simulink model "Backstepping_control"  (R2020b)
settings: Solver=FixedStepAuto  StartTime=0.0  StopTime=500  FixedStep=1e-3  RelTol=1e-3
values from neighbouring files (symbols this model uses):
  g_par = 9.81    [init.m]
  J_par = (M_par*4*l_par^2)/12    (= 192666666.667)    [init.m]
  l_par = 34    [init.m]
  M_par = 5e5    (= 500000)    [init.m]
  mu_x_par = 0.5*rho_par*cdx_par*Ax_par    (= 152.439)    [init.m]
  mu_y_par = 0.5*rho_par*cdy_par*Ay_par    (= 1.28880775561)    [init.m]
  theta0 = deg2rad(15)    [init.m]
  x0 = 2    [init.m]
  y0 = -5    [init.m]
settings Model: Creator=chiara-s  LastModifiedBy=giorg

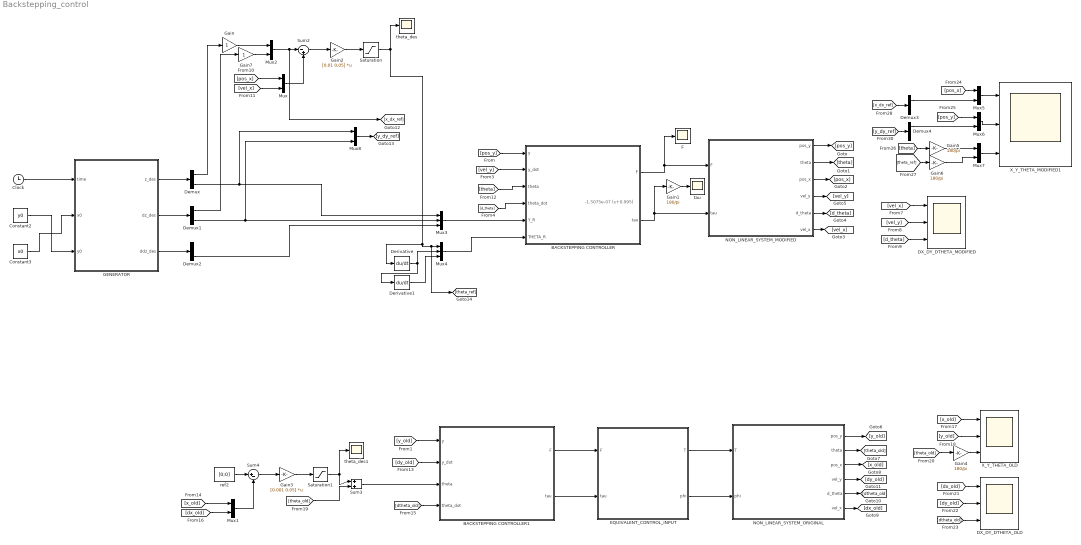
== system Backstepping_control ==
  note: -1.5075e-07 (s+0.995)
  BACKSTEPPING CONTROLLER : Subsystem
  BACKSTEPPING CONTROLLER1 : Subsystem
  Clock : Clock
  Constant2 : Constant  Value=y0
  Constant3 : Constant  Value=x0
  DX_DY_DTHETA_MODIFIED : Scope  NumInputPorts=3
  DX_DY_DTHETA_OLD : Scope  NumInputPorts=3
  Demux{,1..4} (5 alike) : Demux  Outputs=2
  Derivative : Derivative
  Derivative1 : Derivative
  EQUIVALENT_CONTROL_INPUT : MATLAB Function  TreatAsAtomicUnit=on
  F : Scope
  GENERATOR : MATLAB Function  TreatAsAtomicUnit=on
  Gain : Gain
  Gain{1,4..6} (4 alike) : Gain  Gain=180/pi
  Gain2 : Gain  Gain=[0.01 0.05]  Multiplication=Matrix(K*u)
  Gain3 : Gain  Gain=[0.001 0.05]  Multiplication=Matrix(K*u)
  Gain7 : Gain
  Mux{,1..2,5..8} (7 alike) : Mux  Inputs=2
  Mux3 : Mux  Inputs=3
  Mux4 : Mux  Inputs=3
  NON_LINEAR_SYSTEM_MODIFIED : Subsystem
  NON_LINEAR_SYSTEM_ORIGINAL : Subsystem
  Saturation : Saturate  UpperLimit=0.2  LowerLimit=-0.2
  Saturation1 : Saturate  UpperLimit=0.2  LowerLimit=-0.2
  Sum2 : Sum  Inputs=|-+
  Sum3 : Sum  Inputs=|++
  Sum4 : Sum  Inputs=|+-
  X_Y_THETA_MODIFIED1 : Scope  NumInputPorts=3
  X_Y_THETA_OLD : Scope  NumInputPorts=3
  ref2 : Constant  Value=[0;0]
  tau : Scope
  theta_des : Scope
  theta_des1 : Scope
  wires:
  NON_LINEAR_SYSTEM_MODIFIED/1(pos_y) -> [pos_y]
  NON_LINEAR_SYSTEM_MODIFIED/2(theta) -> [theta]
  NON_LINEAR_SYSTEM_MODIFIED/3(pos_x) -> [pos_x]
  NON_LINEAR_SYSTEM_MODIFIED/4(vel_y) -> [vel_y]
  NON_LINEAR_SYSTEM_MODIFIED/5(d_theta) -> [d_theta]
  NON_LINEAR_SYSTEM_MODIFIED/6(vel_x) -> [vel_x]
  [d_theta] -> BACKSTEPPING CONTROLLER/4(theta_dot)
  [pos_y] -> BACKSTEPPING CONTROLLER/1(y)
  [vel_y] -> BACKSTEPPING CONTROLLER/2(y_dot)
  BACKSTEPPING CONTROLLER/1(F) -> NON_LINEAR_SYSTEM_MODIFIED/1(F), F/1
  BACKSTEPPING CONTROLLER/2(tau) -> Gain1/1, NON_LINEAR_SYSTEM_MODIFIED/2(tau)
  [vel_x] -> DX_DY_DTHETA_MODIFIED/1
  [vel_y] -> DX_DY_DTHETA_MODIFIED/2
  [d_theta] -> DX_DY_DTHETA_MODIFIED/3
  Gain1/1 -> tau/1
  Gain2/1 -> Saturation/1
  Mux2/1 -> [x_dx_ref], Sum2/1
  Sum2/1 -> Gain2/1
  Mux/1 -> Sum2/2
  [pos_x] -> Mux/1
  [vel_x] -> Mux/2
  NON_LINEAR_SYSTEM_ORIGINAL/3(pos_x) -> [x_old]
  NON_LINEAR_SYSTEM_ORIGINAL/1(pos_y) -> [y_old]
  NON_LINEAR_SYSTEM_ORIGINAL/4(vel_y) -> [dy_old]
  NON_LINEAR_SYSTEM_ORIGINAL/5(d_theta) -> [dtheta_old]
  NON_LINEAR_SYSTEM_ORIGINAL/2(theta) -> [theta_old]
  NON_LINEAR_SYSTEM_ORIGINAL/6(vel_x) -> [dx_old]
  BACKSTEPPING CONTROLLER1/1(F) -> EQUIVALENT_CONTROL_INPUT/1(F)
  BACKSTEPPING CONTROLLER1/2(tau) -> EQUIVALENT_CONTROL_INPUT/2(tau)
  EQUIVALENT_CONTROL_INPUT/1(T) -> NON_LINEAR_SYSTEM_ORIGINAL/1(T)
  EQUIVALENT_CONTROL_INPUT/2(phi) -> NON_LINEAR_SYSTEM_ORIGINAL/2(phi)
  [y_old] -> BACKSTEPPING CONTROLLER1/1(y)
  [dy_old] -> BACKSTEPPING CONTROLLER1/2(y_dot)
  [dtheta_old] -> BACKSTEPPING CONTROLLER1/4(theta_dot)
  ref2/1 -> Sum4/1
  Sum3/1 -> BACKSTEPPING CONTROLLER1/3(theta)
  [theta_old] -> Sum3/2
  Sum4/1 -> Gain3/1
  [dx_old] -> Mux1/2
  [x_old] -> Mux1/1
  Mux1/1 -> Sum4/2
  Gain3/1 -> Saturation1/1
  Saturation1/1 -> theta_des1/1, Sum3/1
  [x_old] -> X_Y_THETA_OLD/1
  [y_old] -> X_Y_THETA_OLD/2
  [theta_old] -> Gain4/1
  [dx_old] -> DX_DY_DTHETA_OLD/1
  [dy_old] -> DX_DY_DTHETA_OLD/2
  [dtheta_old] -> DX_DY_DTHETA_OLD/3
  Gain4/1 -> X_Y_THETA_OLD/3
  Mux3/1 -> BACKSTEPPING CONTROLLER/5(Y_R)
  Clock/1 -> GENERATOR/1(time)
  Constant2/1 -> GENERATOR/3(y0)
  Constant3/1 -> GENERATOR/2(x0)
  [theta] -> BACKSTEPPING CONTROLLER/3(theta)
  GENERATOR/3(ddz_des) -> Demux2/1
  GENERATOR/2(dz_des) -> Demux1/1
  GENERATOR/1(z_des) -> Demux/1
  Mux4/1 -> BACKSTEPPING CONTROLLER/6(THETA_R)
  Gain6/1 -> Mux7/2
  Mux7/1 -> X_Y_THETA_MODIFIED1/3
  [theta_ref] -> Gain6/1
  Gain5/1 -> Mux7/1
  [x_dx_ref] -> Demux3/1
  Mux6/1 -> X_Y_THETA_MODIFIED1/2
  [pos_x] -> Mux5/1
  Demux3/1 -> Mux5/2
  [pos_y] -> Mux6/1
  [theta] -> Gain5/1
  Mux5/1 -> X_Y_THETA_MODIFIED1/1
  Demux4/1 -> Mux6/2
  [y_dy_ref] -> Demux4/1
  Saturation/1 -> theta_des/1, [theta_ref], Mux4/1, Derivative/1
  Demux/1 -> Gain/1
  Demux1/1 -> Gain7/1
  Derivative/1 -> Mux4/2, Derivative1/1
  Demux/2 -> Mux8/1, Mux3/1
  Demux1/2 -> Mux8/2, Mux3/2
  Demux2/2 -> Mux3/3
  Mux8/1 -> [y_dy_ref]
  Gain/1 -> Mux2/1
  Gain7/1 -> Mux2/2
  Derivative1/1 -> Mux4/3

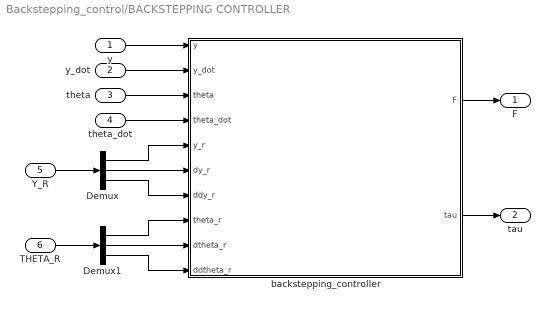
== system Backstepping_control/BACKSTEPPING CONTROLLER ==
  y : Inport
  y_dot : Inport  Port=2
  theta : Inport  Port=3
  theta_dot : Inport  Port=4
  Y_R : Inport  Port=5
  THETA_R : Inport  Port=6
  Demux : Demux  Outputs=3
  Demux1 : Demux  Outputs=3
  backstepping_controller : MATLAB Function  TreatAsAtomicUnit=on
  F : Outport
  tau : Outport  Port=2
  wires:
  backstepping_controller/1(F) -> F/1
  backstepping_controller/2(tau) -> tau/1
  y/1 -> backstepping_controller/1(y)
  y_dot/1 -> backstepping_controller/2(y_dot)
  theta/1 -> backstepping_controller/3(theta)
  theta_dot/1 -> backstepping_controller/4(theta_dot)
  Demux/1 -> backstepping_controller/5(y_r)
  Demux/2 -> backstepping_controller/6(dy_r)
  Demux/3 -> backstepping_controller/7(ddy_r)
  Y_R/1 -> Demux/1
  Demux1/2 -> backstepping_controller/9(dtheta_r)
  Demux1/1 -> backstepping_controller/8(theta_r)
  Demux1/3 -> backstepping_controller/10(ddtheta_r)
  THETA_R/1 -> Demux1/1

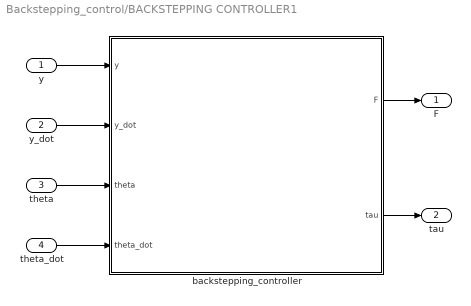
== system Backstepping_control/BACKSTEPPING CONTROLLER1 ==
  y : Inport
  y_dot : Inport  Port=2
  theta : Inport  Port=3
  theta_dot : Inport  Port=4
  backstepping_controller : MATLAB Function  TreatAsAtomicUnit=on
  F : Outport
  tau : Outport  Port=2
  wires:
  backstepping_controller/1(F) -> F/1
  backstepping_controller/2(tau) -> tau/1
  y/1 -> backstepping_controller/1(y)
  y_dot/1 -> backstepping_controller/2(y_dot)
  theta/1 -> backstepping_controller/3(theta)
  theta_dot/1 -> backstepping_controller/4(theta_dot)

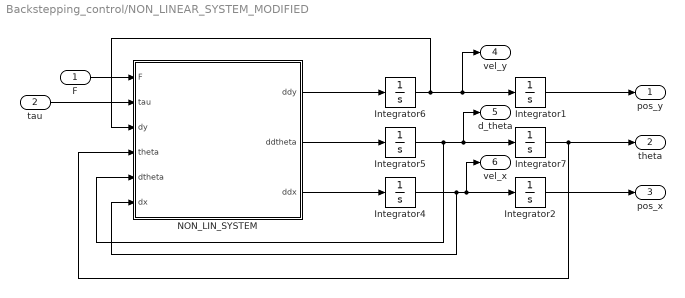
== system Backstepping_control/NON_LINEAR_SYSTEM_MODIFIED ==
  F : Inport
  tau : Inport  Port=2
  Integrator1 : Integrator  InitialCondition=y0
  Integrator2 : Integrator  InitialCondition=x0
  Integrator4 : Integrator
  Integrator5 : Integrator
  Integrator6 : Integrator
  Integrator7 : Integrator  InitialCondition=theta0
  NON_LIN_SYSTEM : MATLAB Function  TreatAsAtomicUnit=on
  pos_y : Outport
  theta : Outport  Port=2
  pos_x : Outport  Port=3
  vel_y : Outport  Port=4
  d_theta : Outport  Port=5
  vel_x : Outport  Port=6
  wires:
  Integrator2/1 -> pos_x/1
  Integrator7/1 -> NON_LIN_SYSTEM/4(theta), theta/1
  NON_LIN_SYSTEM/2(ddtheta) -> Integrator5/1
  tau/1 -> NON_LIN_SYSTEM/2(tau)
  Integrator1/1 -> pos_y/1
  F/1 -> NON_LIN_SYSTEM/1(F)
  Integrator6/1 -> Integrator1/1, vel_y/1, NON_LIN_SYSTEM/3(dy)
  Integrator4/1 -> NON_LIN_SYSTEM/6(dx), vel_x/1, Integrator2/1
  NON_LIN_SYSTEM/1(ddy) -> Integrator6/1
  Integrator5/1 -> NON_LIN_SYSTEM/5(dtheta), Integrator7/1, d_theta/1
  NON_LIN_SYSTEM/3(ddx) -> Integrator4/1

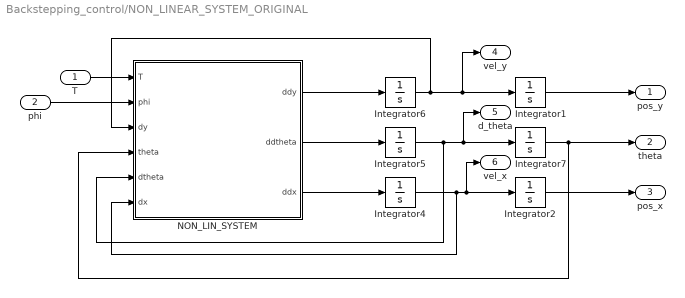
== system Backstepping_control/NON_LINEAR_SYSTEM_ORIGINAL ==
  T : Inport
  phi : Inport  Port=2
  Integrator1 : Integrator  InitialCondition=y0
  Integrator2 : Integrator  InitialCondition=x0
  Integrator4 : Integrator
  Integrator5 : Integrator
  Integrator6 : Integrator
  Integrator7 : Integrator  InitialCondition=theta0
  NON_LIN_SYSTEM : MATLAB Function  TreatAsAtomicUnit=on
  pos_y : Outport
  theta : Outport  Port=2
  pos_x : Outport  Port=3
  vel_y : Outport  Port=4
  d_theta : Outport  Port=5
  vel_x : Outport  Port=6
  wires:
  Integrator2/1 -> pos_x/1
  Integrator7/1 -> NON_LIN_SYSTEM/4(theta), theta/1
  NON_LIN_SYSTEM/2(ddtheta) -> Integrator5/1
  phi/1 -> NON_LIN_SYSTEM/2(phi)
  Integrator1/1 -> pos_y/1
  T/1 -> NON_LIN_SYSTEM/1(T)
  Integrator6/1 -> Integrator1/1, vel_y/1, NON_LIN_SYSTEM/3(dy)
  Integrator4/1 -> NON_LIN_SYSTEM/6(dx), vel_x/1, Integrator2/1
  NON_LIN_SYSTEM/1(ddy) -> Integrator6/1
  Integrator5/1 -> NON_LIN_SYSTEM/5(dtheta), Integrator7/1, d_theta/1
  NON_LIN_SYSTEM/3(ddx) -> Integrator4/1

== matlab function Backstepping_control/GENERATOR ==
  data: time input; x0 input; y0 input; z_des output; dz_des output; ddz_des output
function  [z_des, dz_des, ddz_des] = fcn(time,x0,y0)
t= time;
pos_init = [x0;y0];
z_des = pos_init + [20*sin(0.1*t); 10*sin(0.2*t)];
dz_des = [cos(0.1*t)*2; cos(0.2*t)*2];
ddz_des = [-sin(0.1*t)*0.2; -sin(0.2*t)*0.4];

% pos_init = [y0;theta0];
% z_des = pos_init + [20*sin(0.1*t); 10*pi/180*sin(0.2*t)];
% dz_des = [cos(0.1*t)*2; pi/180*cos(0.2*t)*2];
% ddz_des = [-sin(0.1*t)*0.2; -pi/180*sin(0.2*t)*0.4];
end

== matlab function Backstepping_control/BACKSTEPPING CONTROLLER/backstepping_controller ==
  data: y input; F output; y_dot input; theta input; theta_dot input; y_r input; dy_r input; ddy_r input; theta_r input; dtheta_r input; ddtheta_r input; tau output; g_par parameter; mu_y_par parameter; J_par parameter; M_par parameter
function [F,tau] = fcn(y,y_dot,theta,theta_dot, y_r, dy_r, ddy_r, theta_r, dtheta_r, ddtheta_r, g_par, mu_y_par, J_par, M_par)

% F = M_par*(-2*y_dot - y + g_par + (mu_y_par/M_par)*y_dot)/cos(theta);
% tau = -J_par*(theta + 2*theta_dot);

F = (M_par/cos(theta))*(ddy_r + 2*dy_r + y_r -y_dot*(2-mu_y_par/M_par) - y + g_par);
tau = J_par*(ddtheta_r + 2*dtheta_r + theta_r -2*theta_dot - theta);

end

== matlab function Backstepping_control/NON_LINEAR_SYSTEM_MODIFIED/NON_LIN_SYSTEM ==
  data: F input; ddy output; tau input; dy input; theta input; dtheta input; dx input; ddtheta output; ddx output; M_par parameter; mu_x_par parameter; J_par parameter; l_par parameter; mu_y_par parameter; g_par parameter
function [ddy, ddtheta, ddx] = fcn(F, tau, dy, theta, dtheta, dx, M_par, mu_x_par, J_par, l_par, mu_y_par, g_par)

% u = [F,tau] here we consider alligned thrusther with y axis and torque
% tau 
ddx = M_par^-1*(-F*sin(theta) - mu_x_par*dx);
ddtheta = J_par^-1*tau;
ddy = M_par^-1*(F*cos(theta) - mu_y_par*dy - M_par*g_par);


end

== matlab function Backstepping_control/NON_LINEAR_SYSTEM_ORIGINAL/NON_LIN_SYSTEM ==
  data: T input; ddy output; phi input; dy input; theta input; dtheta input; dx input; ddtheta output; ddx output; M_par parameter; mu_x_par parameter; J_par parameter; l_par parameter; mu_y_par parameter; g_par parameter
function [ddy, ddtheta, ddx] = fcn(T, phi, dy, theta, dtheta, dx, M_par, mu_x_par, J_par, l_par, mu_y_par, g_par)

ddx = M_par^-1*(-T*sin(theta+phi) - mu_x_par*dx);
ddtheta = J_par^-1*(-T*l_par*sin(phi));
ddy = M_par^-1*(T*cos(theta+phi) - mu_y_par*dy - M_par*g_par);


end

== matlab function Backstepping_control/BACKSTEPPING CONTROLLER1/backstepping_controller ==
  data: y input; F output; y_dot input; theta input; theta_dot input; tau output; g_par parameter; mu_y_par parameter; J_par parameter; M_par parameter
function [F,tau] = fcn(y,y_dot,theta,theta_dot, g_par, mu_y_par, J_par, M_par)


F = M_par*(-2*y_dot - y + g_par + (mu_y_par/M_par)*y_dot)/cos(theta);
tau = -J_par*(theta + 2*theta_dot);

end

== matlab function Backstepping_control/EQUIVALENT_CONTROL_INPUT ==
  data: F input; T output; tau input; phi output; l_par parameter
function [T, phi] = fcn(F,tau, l_par)

phi = -atan2(tau,F*l_par);
T = F/cos(phi);



end
